simulink model "Test"  (R2023b)
settings: Solver=VariableStepAuto  StartTime=0.0  StopTime=30  RelTol=1e-3
settings Model: Creator=MrLove  LastModifiedBy=MrLove

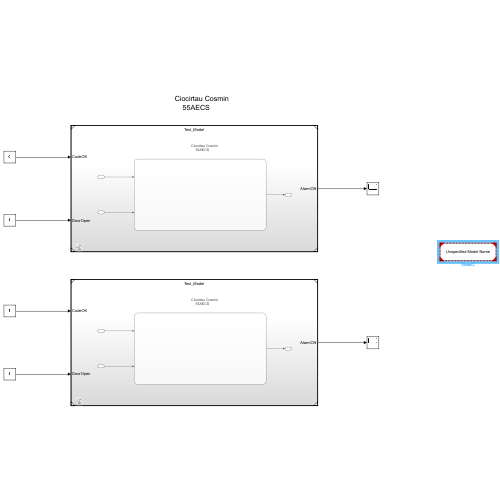
[thumbnail: Simulink's stored preview of the top-level diagram]
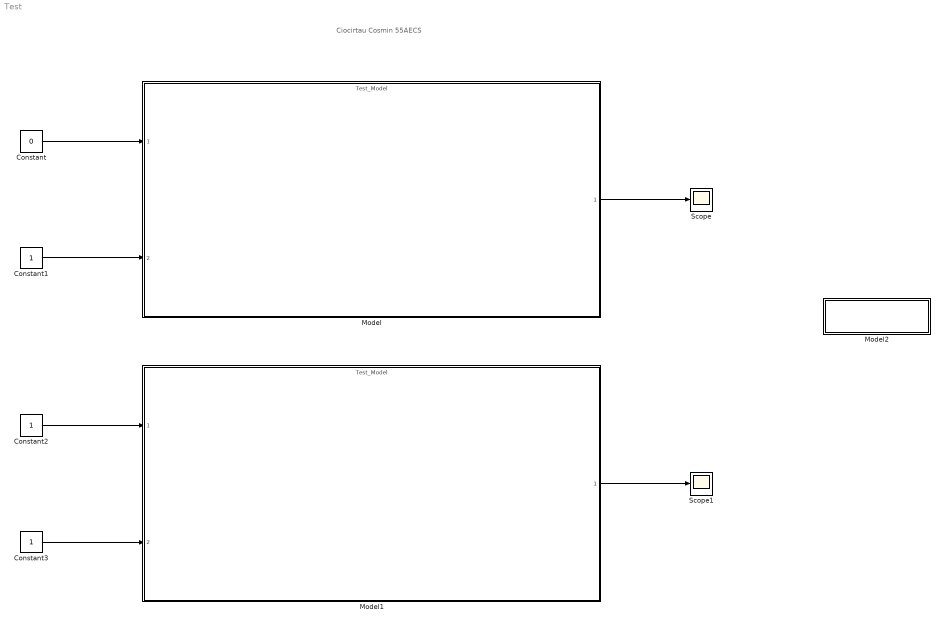
== system Test ==
  note: Ciocirtau Cosmin
      | 55AECS
  Constant : Constant  Value=0
  Constant1 : Constant
  Constant2 : Constant
  Constant3 : Constant
  Model : ModelReference  ModelNameDialog=Test_Model.slx  SimulationMode=Normal  ModelReferenceVersion=1.5
  Model1 : ModelReference  ModelNameDialog=Test_Model.slx  SimulationMode=Normal  ModelReferenceVersion=1.5
  Model2 : ModelReference  SimulationMode=Normal
  Scope : Scope
  Scope1 : Scope
  wires:
  Constant/1 -> Model/1
  Constant1/1 -> Model/2
  Model/1 -> Scope/1
  Constant2/1 -> Model1/1
  Constant3/1 -> Model1/2
  Model1/1 -> Scope1/1
